simulink model "soc_swhw_proc"  (R2021a)
settings: Solver=FixedStepDiscrete  StartTime=0.0  StopTime=10.0  RelTol=1e-3  EnableMultiTasking=on
PreLoadFcn:
  | hsb.blkcb2.defineTypes;
  | if exist('sampleTime') ~=1
  | FrameSize = 8192;
  | sampleTime = 0.1e-6;
  | NumBuffers = 4;
  | end
libraries: prociolib x2, simulink x1
settings Model: Creator=The MathWorks, Inc.  LastModifiedBy=AliReza
settings SolverCC: ConcurrentTasks=on  AlgebraicLoopSolver=TrustRegion  PositivePriorityOrder=on  InsertRTBMode=Never (minimum delay)
settings DataIOCC: SaveFormat=StructureWithTime  ReturnWorkspaceOutputs=off
settings OptimizationCC: EnhancedBackFolding=on  PassReuseOutputArgsAs=Individual arguments  ZeroExternalMemoryAtStartup=off  MaxStackSize=64  OptimizeBlockOrder=speed  DifferentSizesBufferReuse=on  OptimizationCustomize=off  EfficientTunableParamExpr=on
settings DebuggingCC: IntegerOverflowMsg=none  ParameterTunabilityLossMsg=error  SFMachineParentedDataDiag=warning  ArithmeticOperatorsInVariantConditions=warning
settings HardwareCC: ProdBitPerPointer=32  ProdBitPerSizeT=32  ProdBitPerPtrDiffT=32  ProdLargestAtomicInteger=Long  ProdLargestAtomicFloat=Double  ProdWordSize=32  ProdLongLongMode=on  ProdHWDeviceType=ARM Compatible->ARM Cortex  HardwareBoardFeatureSet=SoCBlockset
settings ModelReferenceCC: ModelReferenceNumInstancesAllowed=Single
settings SFSimCC: SimUseLocalCustomCode=off  MATLABDynamicMemAlloc=off
settings RTWCC: SystemTargetFile=ert.tlc  HardwareBoard=Altera Cyclone V SoC development kit  TLCOptions="-aInlineSetEventsForThisBaseRateFcn=TLC_FALSE -aSuppressMultiTaskScheduler=TLC_FALSE  -aRateBasedStepFcn=0"  TemplateMakefile=ert_default_tmf  GenerateReport=on  RTWUseLocalCustomCode=off  Toolchain=ARM Development Studio Altera Edition (DS-5 AE)  IncludeHyperlinkInReport=on  LaunchReport=on  GenerateTraceInfo=on  GenerateTraceReport=on  GenerateTraceReportSl=on  GenerateTraceReportSf=on  GenerateTraceReportEml=on
settings CodeAppCC: ForceParamTrailComments=on  IgnoreCustomStorageClasses=off  OperatorAnnotations=on  SimulinkDataObjDesc=on  SFDataObjDesc=on  InsertBlockDesc=on

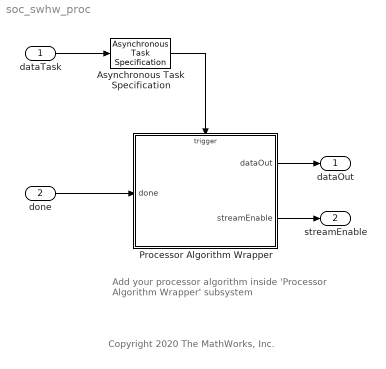
== system soc_swhw_proc ==
  note: Add your processor algorithm inside
      | 'Processor Algorithm Wrapper' subsystem
  note: Copyright 2020 The MathWorks, Inc.
  dataTask : Inport  OutputFunctionCall=on
  done : Inport  OutputPortMessageModes=m  Port=2  OutDataTypeStr=boolean  BusOutputAsStruct=on
  Asynchronous Task Specification : AsynchronousTaskSpecification  TaskPriority=50
  Processor Algorithm Wrapper : Subsystem  TreatAsAtomicUnit=on
  dataOut : Outport  VectorParamsAs1DForOutWhenUnconnected=off
  streamEnable : Outport  Port=2
  wires:
  dataTask/1 -> Asynchronous Task Specification/1
  Processor Algorithm Wrapper/1(dataOut) -> dataOut/1
  done/1 -> Processor Algorithm Wrapper/1(done)
  Asynchronous Task Specification/1 -> Processor Algorithm Wrapper/Trigger
  Processor Algorithm Wrapper/2(streamEnable) -> streamEnable/1

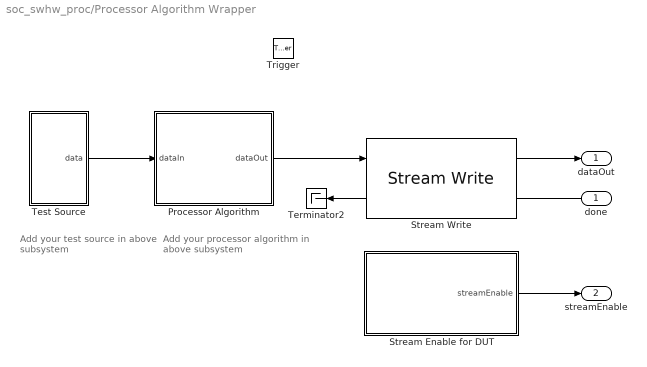
== system soc_swhw_proc/Processor Algorithm Wrapper ==
  note: Add your processor algorithm
      | in above subsystem
  note: Add your test source
      | in above subsystem
  done : Inport
  Trigger : TriggerPort  TriggerType=function-call  VariantControl=Variant  PortDimensions=1
  Processor Algorithm : Subsystem
  Stream Enable for DUT : Subsystem
  Stream Write : prociolib/Stream Write  DeviceName=mwipcore0:mm2s  NumberOfBuffers=NumBuffers  EnableEvent=on
      settings: SourceProductBaseCode=HW
  Terminator2 : Terminator
  Test Source : Subsystem
  dataOut : Outport  VectorParamsAs1DForOutWhenUnconnected=off
  streamEnable : Outport  Port=2
  wires:
  done/1 -> Stream Write/2
  Stream Write/1 -> dataOut/1
  Stream Write/2 -> Terminator2/1
  Processor Algorithm/1(dataOut) -> Stream Write/1
  Test Source/1(data) -> Processor Algorithm/1(dataIn)
  Stream Enable for DUT/1(streamEnable) -> streamEnable/1

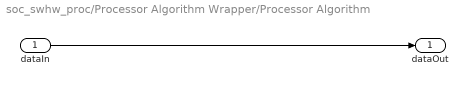
== system soc_swhw_proc/Processor Algorithm Wrapper/Processor Algorithm ==
  dataIn : Inport
  dataOut : Outport  VectorParamsAs1DForOutWhenUnconnected=off
  wires:
  dataIn/1 -> dataOut/1

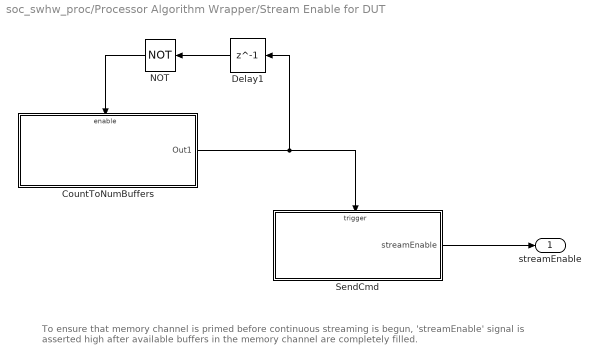
== system soc_swhw_proc/Processor Algorithm Wrapper/Stream Enable for DUT ==
  note: To ensure that memory channel is primed before continuous streaming is begun,
      | 'streamEnable' signal is asserted high after available buffers in the memory channel are completely filled.
  CountToNumBuffers : Subsystem
  Delay1 : Delay  DelayLength=1  InitialCondition=0
  NOT : Logic  Operator=NOT  AllPortsSameDT=off  OutDataTypeStr=boolean
  SendCmd : Subsystem
  streamEnable : Outport
  wires:
  SendCmd/1(streamEnable) -> streamEnable/1
  Delay1/1 -> NOT/1
  CountToNumBuffers/1(Out1) -> SendCmd/Trigger, Delay1/1
  NOT/1 -> CountToNumBuffers/Enable

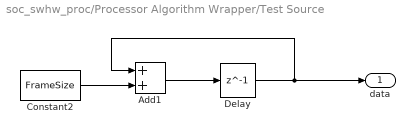
== system soc_swhw_proc/Processor Algorithm Wrapper/Test Source ==
  Add1 : Sum  AccumDataTypeStr=uint32  OutDataTypeStr=uint32
  Constant2 : Constant  Value=FrameSize  OutDataTypeStr=uint32  SampleTime=-1
  Delay : Delay  DelayLength=1  InitialCondition=uint32([0:FrameSize-1])
  data : Outport
  wires:
  Delay/1 -> data/1, Add1/1
  Constant2/1 -> Add1/2
  Add1/1 -> Delay/1

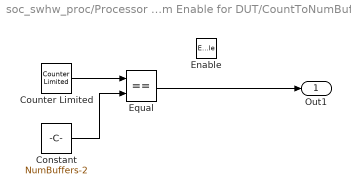
== system soc_swhw_proc/Processor Algorithm Wrapper/Stream Enable for DUT/CountToNumBuffers ==
  Enable : EnablePort
  Constant : Constant  Value=NumBuffers-2  SampleTime=-1
  Counter Limited : simulink/Sources/Counter Limited  uplimit=NumBuffers-2  tsamp=-1
  Equal : RelationalOperator  Operator===  OutDataTypeStr=boolean  RndMeth=Simplest
  Out1 : Outport
  wires:
  Counter Limited/1 -> Equal/1
  Constant/1 -> Equal/2
  Equal/1 -> Out1/1

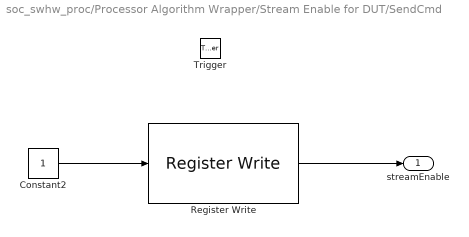
== system soc_swhw_proc/Processor Algorithm Wrapper/Stream Enable for DUT/SendCmd ==
  Trigger : TriggerPort  VariantControl=Variant  PortDimensions=1
  Constant2 : Constant  OutDataTypeStr=boolean  SampleTime=-1
  Register Write : prociolib/Register Write  OutputSink=To output port  TunableParamName=A  RegisterName=RegA  DeviceName=/dev/mwipcore  OffsetAddress=hex2dec('100')  Dummy=0
      settings: SourceProductBaseCode=HW
  streamEnable : Outport
  wires:
  Constant2/1 -> Register Write/1
  Register Write/1 -> streamEnable/1
